simulink model "sl_groundvehicleDynamics"  (R2025a)
settings: Solver=ode45  StartTime=0.0  StopTime=1500  RelTol=1e-5  EnableMultiTasking=on
InitFcn:
  | mdl_robot;
undefined symbols (not defined in the file or in its folder): robot, waypoints
libraries: simulink x4, mobileRoboticsLib x3, simulink_extras x2
settings Model: Creator=sriramn  LastModifiedBy=n10971327
settings SolverCC: ZeroCrossAlgorithm=Adaptive  AlgebraicLoopSolver=TrustRegion
settings DataIOCC: LimitDataPoints=on  SaveFormat=Array  ReturnWorkspaceOutputs=off
settings OptimizationCC: ReuseModelBlockBuffer=off  LifeSpan=inf
settings DebuggingCC: SolverPrmCheckMsg=warning  UnconnectedInputMsg=warning  UnconnectedOutputMsg=warning  UnconnectedLineMsg=warning  AllowSymbolicDim=off  SFUnexpectedBacktrackingDiag=warning  SFNoUnconditionalDefaultTransitionDiag=warning  SFExecutionAtInitializationDiag=none  ArithmeticOperatorsInVariantConditions=warning
settings HardwareCC: ProdBitPerPointer=32.0  ProdBitPerSizeT=32.0  ProdBitPerPtrDiffT=32.0  ProdLargestAtomicFloat=None  ProdIntDivRoundTo=Undefined  ProdEndianess=Unspecified  ProdWordSize=32.0  ProdHWDeviceType=32-bit Generic
settings ModelReferenceCC: EnableRefExpFcnMdlSchedulingChecks=on  ModelReferenceMinAlgLoopOccurrences=on  PropagateSignalLabelsOutOfModel=off
settings SFSimCC: SimUseLocalCustomCode=off  CustomCodeUndefinedFunction=UseInterfaceOnly
settings RTWCC: RTWUseLocalCustomCode=off  GPUComputeCapability=3.5
settings CodeAppCC: StateflowObjectComments=on
settings GRTTargetCC: TargetLangStandard=C89/C90 (ANSI)
settings ConfigComp: CovMetricSettings=dw  CovSaveCumulativeToWorkspaceVar=on  CovSaveSingleToWorkspaceVar=on  CovExternalEMLEnable=off  CovSFcnEnable=off
settings SimscapeCC: SimscapeNormalizeSystem=off
settings ConfigurationSet: Description=SimMechanics 2G
settings ExplorerConfigSet: InternalSimMechanicsExplorerSettings="<ExplorerConfiguration><canonicalview>planar_xy</canonicalview><AnimationSetting><BasePlaybackSpeed>1.0</BasePlaybackSpeed><PlaybackSpeedFactor>1.0</PlaybackSpeedFactor></AnimationSetting><TilePanel><TileInfo><Tiles Columns=\"1\" Count=\"1\" Rows=\"1\"><Column Left=\"2\" Weight=\"1\"/><Column Left=\"1628\"/><Row Top=\"2\" Weight=\"1\"/><Row Top=\"1072\"/><Tile Height=\"1\" Width=\"1\" X=\"0\" Y=\"0\"/></Tiles></TileInfo><SceneInfo><SceneViewer><BGColor><R>0.60000002384185791</R><G>0.60000002384185791</G><B>0.60000002384185791</B></BGColor><Camera><Position><X>0.22951840878551699</X><Y>0.32651610611526627</Y><Z>-0.27215421354393321</Z></Position><Center><X>-0.15775714411666431</X><Y>-0.15462825985839526</Y><Z>0.065702552916005602</Z></Center><Up><X>-0.56030137557930915</X><Y>0.72817587161684794</Y><Z>0.39474329445726858</Z></Up><Left>-0.21481383955700509</Left><Right>0.21481383955700509</Right><Bottom>-0.27569784609469139</Bottom><Top>0.27569784609469139</Top></Camera></SceneViewer></SceneInfo></TilePanel></ExplorerConfiguration>"

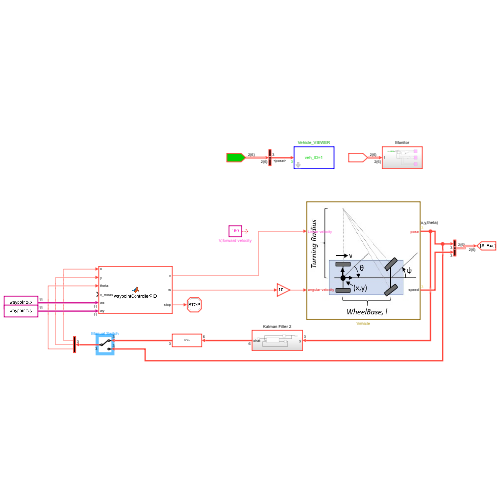
[thumbnail: Simulink's stored preview of the top-level diagram]
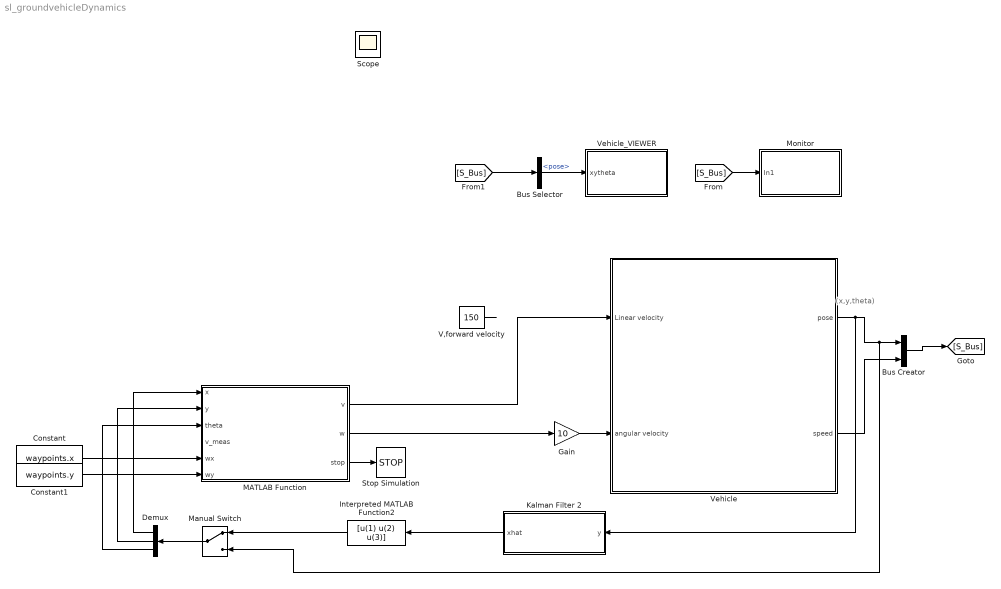
== system sl_groundvehicleDynamics ==
  note: (x,y,theta)
  Bus Creator : BusCreator  Inputs=2
  Bus Selector : BusSelector  OutputSignals=pose
  Constant : Constant  Value=waypoints.x
  Constant1 : Constant  Value=waypoints.y
  Demux : Demux  Outputs=3
  Gain : Gain  Gain=10
  Interpreted MATLAB Function2 : MATLABFcn  MATLABFcn=[u(1) u(2) u(3)]
  Kalman Filter 2 : Subsystem
  MATLAB Function : MATLAB Function  TreatAsAtomicUnit=on
  Manual Switch : ManualSwitch
  Monitor : Subsystem
  Stop Simulation : Stop
  V,forward velocity : Constant  Value=150
  Vehicle : Subsystem
      mask Display: image('vehicle.jpg');
  Vehicle_VIEWER : Subsystem  mask{wp_mat=[waypoints.x(:), waypoints.y(:)], veh_ID_num=1, veh_init_xytheta=[robot.X robot.Y robot.Theta], Ts=0.5}
      mask prompts: wp_mat "Waypoint matrix for arena [x_col, y_col] (m)"; veh_ID_num "Vehicle ID number"; veh_init_xytheta "Initial pose [x,y,theta]"; Ts "Sample time for updating animation (secs)"
      mask TypeOptions veh_ID_num: 1 | 2 | 3 | 4
      mask DialogControl Control2 Prompt: Animate simulation of Differential Drive Robot (DDR)
      mask Display: fprintf('veh_ID=%d',veh_ID_num);
  Scope : Scope
      settings: ActiveDisplayYMinimum=0.07  ActiveDisplayYMaximum=0.09
  wires:
  [S_Bus] -> Monitor/1(In1)
  [S_Bus] -> Bus Selector/1
  Vehicle/1(pose) -> Kalman Filter 2/1(y), Manual Switch/2, Bus Creator/1
  Vehicle/2(speed) -> Bus Creator/2
  Bus Creator/1 -> [S_Bus]
  Bus Selector/1 -> Vehicle_VIEWER/1(xytheta)  "<pose>"
  MATLAB Function/2(w) -> Gain/1
  V,forward velocity/1 -> ?
  Gain/1 -> Vehicle/2(angular velocity)
  MATLAB Function/3(stop) -> Stop Simulation/1
  Constant/1 -> MATLAB Function/5(wx)
  Constant1/1 -> MATLAB Function/6(wy)
  MATLAB Function/1(v) -> Vehicle/1(Linear velocity)
  Kalman Filter 2/1(xhat) -> Interpreted MATLAB Function2/1
  Demux/1 -> MATLAB Function/1(x)
  Interpreted MATLAB Function2/1 -> Manual Switch/1
  Manual Switch/1 -> Demux/1
  Demux/2 -> MATLAB Function/2(y)
  Demux/3 -> MATLAB Function/3(theta)

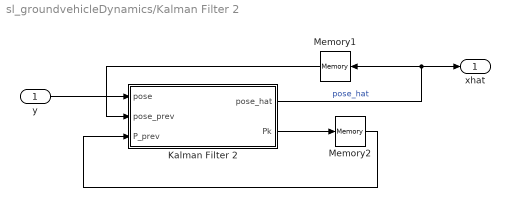
== system sl_groundvehicleDynamics/Kalman Filter 2 ==
  y : Inport
  Kalman Filter 2 : MATLAB Function  TreatAsAtomicUnit=on
  Memory1 : Memory  InheritSampleTime=on
  Memory2 : Memory  InheritSampleTime=on
  xhat : Outport
  wires:
  y/1 -> Kalman Filter 2/1(pose)
  Memory1/1 -> Kalman Filter 2/2(pose_prev)
  Kalman Filter 2/2(Pk) -> Memory2/1
  Kalman Filter 2/1(pose_hat) -> xhat/1, Memory1/1  "pose_hat"
  Memory2/1 -> Kalman Filter 2/3(P_prev)

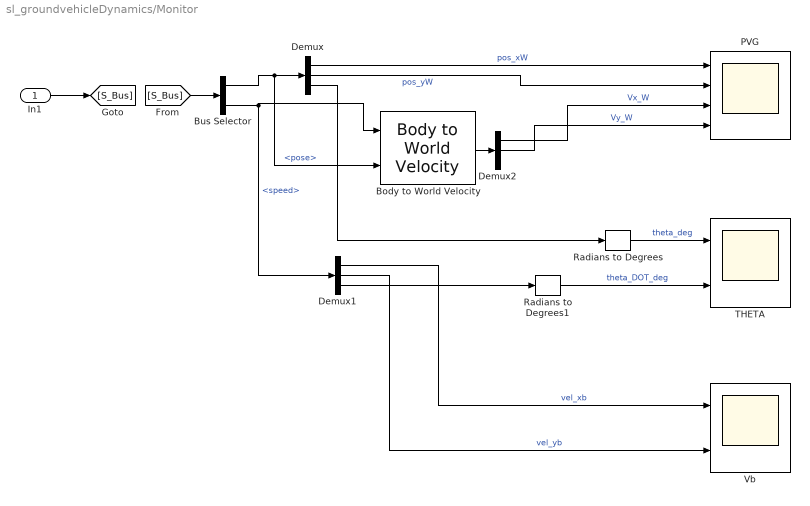
== system sl_groundvehicleDynamics/Monitor ==
  In1 : Inport
  Body to World Velocity : mobileRoboticsLib/Utilities/Body to World Velocity
      settings: SourceProductName=Mobile Robotics Simulation Toolbox
  Bus Selector : BusSelector  OutputSignals=pose,speed
  Demux : Demux  Outputs=3
  Demux1 : Demux  Outputs=3
  Demux2 : Demux  Outputs=3
  PVG : Scope  NumInputPorts=4
      settings: ActiveDisplayYMinimum=-3.02358  ActiveDisplayYMaximum=27.35477
  Radians to Degrees : simulink_extras/Transformations/Radians to Degrees
  Radians to Degrees1 : simulink_extras/Transformations/Radians to Degrees
  THETA : Scope  NumInputPorts=2
      settings: ActiveDisplayYMinimum=-8.72937  ActiveDisplayYMaximum=60.06611  DataLoggingVariableName=ScopeData2
  Vb : Scope  NumInputPorts=2
      settings: ActiveDisplayYMinimum=0.05577  ActiveDisplayYMaximum=0.8929
  wires:
  In1/1 -> [S_Bus]
  [S_Bus] -> Bus Selector/1
  Demux/1 -> PVG/1  "pos_xW"
  Demux/2 -> PVG/2  "pos_yW"
  Radians to Degrees1/1 -> THETA/2  "theta_DOT_deg"
  Radians to Degrees/1 -> THETA/1  "theta_deg"
  Demux1/3 -> Radians to Degrees1/1
  Demux/3 -> Radians to Degrees/1
  Bus Selector/1 -> Body to World Velocity/2, Demux/1  "<pose>"
  Bus Selector/2 -> Demux1/1, Body to World Velocity/1  "<speed>"
  Body to World Velocity/1 -> Demux2/1
  Demux2/1 -> PVG/3  "Vx_W"
  Demux2/2 -> PVG/4  "Vy_W"
  Demux1/1 -> Vb/1  "vel_xb"
  Demux1/2 -> Vb/2  "vel_yb"

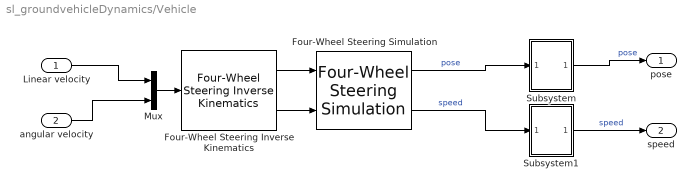
== system sl_groundvehicleDynamics/Vehicle ==
  Linear velocity : Inport
  angular velocity : Inport  Port=2
  Four-Wheel Steering Inverse Kinematics : mobileRoboticsLib/Kinematic Models/Four-Wheel Steering/Four-Wheel Steering Inverse Kinematics  wheelRadius=0.1  frontWheelDist=0.25  rearWheelDist=0.25  ikMode=Front Steering
      settings: SourceProductName=Mobile Robotics Simulation Toolbox
  Four-Wheel Steering Simulation : mobileRoboticsLib/Kinematic Models/Four-Wheel Steering/Four-Wheel Steering Simulation  wheelRadius=0.1  frontWheelDist=0.25  rearWheelDist=0.25  initX=robot.X  initY=robot.Y  initAngle=robot.Theta  Ts=0.05
      settings: SourceProductName=Mobile Robotics Simulation Toolbox
  Mux : Mux  Inputs=2
  Subsystem : Subsystem
  Subsystem1 : Subsystem
  pose : Outport  VectorParamsAs1DForOutWhenUnconnected=off
  speed : Outport  Port=2
  wires:
  angular velocity/1 -> Mux/2
  Linear velocity/1 -> Mux/1
  Mux/1 -> Four-Wheel Steering Inverse Kinematics/1
  Four-Wheel Steering Simulation/1 -> Subsystem/1(In1)  "pose"
  Four-Wheel Steering Simulation/2 -> Subsystem1/1(In1)  "speed"
  Four-Wheel Steering Inverse Kinematics/1 -> Four-Wheel Steering Simulation/1
  Four-Wheel Steering Inverse Kinematics/2 -> Four-Wheel Steering Simulation/2
  Subsystem/1(pose) -> pose/1  "pose"
  Subsystem1/1(speed) -> speed/1  "speed"

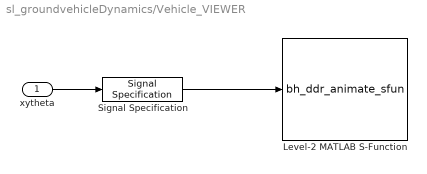
== system sl_groundvehicleDynamics/Vehicle_VIEWER ==
  xytheta : Inport
  Level-2 MATLAB S-Function : M-S-Function  FunctionName=bh_ddr_animate_sfun  Parameters=Ts, wp_mat, veh_ID_num, veh_init_xytheta
  Signal Specification : SignalSpecification  Dimensions=3
  wires:
  xytheta/1 -> Signal Specification/1
  Signal Specification/1 -> Level-2 MATLAB S-Function/1

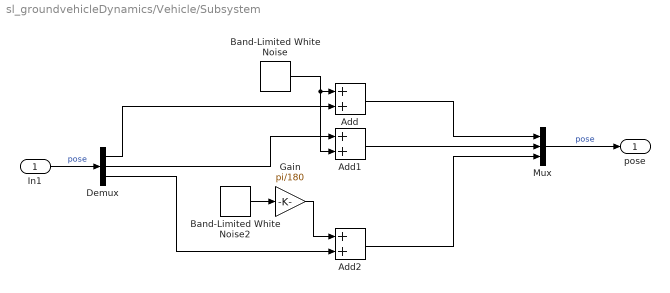
== system sl_groundvehicleDynamics/Vehicle/Subsystem ==
  In1 : Inport
  Add : Sum
  Add1 : Sum
  Add2 : Sum
  Band-Limited White Noise : simulink/Sources/Band-Limited White Noise  Cov=[0.001]  Ts=0.1  seed=[23341]
  Band-Limited White Noise2 : simulink/Sources/Band-Limited White Noise  Cov=[0.41]  Ts=0.1  seed=[23341]
  Demux : Demux  Outputs=3
  Gain : Gain  Gain=pi/180
  Mux : Mux  Inputs=3
  pose : Outport
  wires:
  Add1/1 -> Mux/2
  Add2/1 -> Mux/3
  Demux/2 -> Add1/1
  Band-Limited White Noise2/1 -> Gain/1
  Demux/3 -> Add2/2
  Band-Limited White Noise/1 -> Add1/2, Add/1
  In1/1 -> Demux/1  "pose"
  Demux/1 -> Add/2
  Gain/1 -> Add2/1
  Mux/1 -> pose/1  "pose"
  Add/1 -> Mux/1

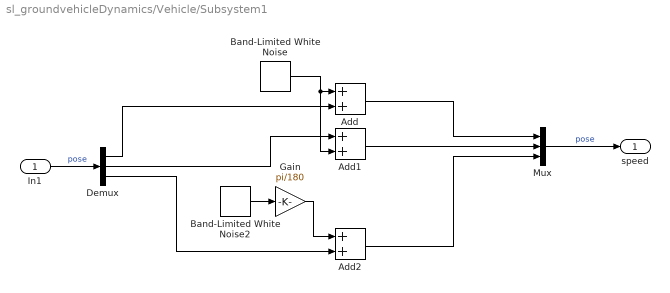
== system sl_groundvehicleDynamics/Vehicle/Subsystem1 ==
  In1 : Inport
  Add : Sum
  Add1 : Sum
  Add2 : Sum
  Band-Limited White Noise : simulink/Sources/Band-Limited White Noise  Cov=[0.001]  Ts=0.1  seed=[23341]
  Band-Limited White Noise2 : simulink/Sources/Band-Limited White Noise  Cov=[0.41]  Ts=0.1  seed=[23341]
  Demux : Demux  Outputs=3
  Gain : Gain  Gain=pi/180
  Mux : Mux  Inputs=3
  speed : Outport
  wires:
  Add1/1 -> Mux/2
  Add2/1 -> Mux/3
  Demux/2 -> Add1/1
  Band-Limited White Noise2/1 -> Gain/1
  Demux/3 -> Add2/2
  Band-Limited White Noise/1 -> Add1/2, Add/1
  In1/1 -> Demux/1  "pose"
  Demux/1 -> Add/2
  Gain/1 -> Add2/1
  Mux/1 -> speed/1  "pose"
  Add/1 -> Mux/1

== matlab function sl_groundvehicleDynamics/MATLAB Function ==
  data: v output; x input; w output; y input; theta input; v_meas input; wx input; wy input; stop output
function [v, w, stop] = waypointControllerPID(x, y, theta, v_meas, wx, wy)
%% Tuning Variables
% Controller sample time (s) – set to your model's controller step
Ts = 0.02;

% Heading PID (for w)
Kp_h = 1.6;     Ki_h = 0.20;   Kd_h = 0.05;
w_max = 1.2;                  % [rad/s] limit
i_lim_h = 2.0;                % integral clamp

% Speed PI (for v)
Kp_v = 1.0;     Ki_v = 0.5;
v_max = 100;   v_min = 0.0;   % [m/s]
i_lim_v = 5.0;

% Waypoint logic
capture_R   = 5.0;            % [m] switch waypoint
slow_R      = 40.0;           % [m] start slowing down near wp
e_slow_max  = pi/2;           % slow for big heading error (≈90°)

% Cruise bias (regular speed)
v_cruise    = 20;            % [m/s]
%% 

wx = wx(:);
wy = wy(:);
N  = numel(wx);

% Persistent state
persistent idx ih iv eh_prev Nprev
if isempty(idx);     idx = 1;        end
if isempty(ih);      ih  = 0.0;      end
if isempty(iv);      iv  = 0.0;      end
if isempty(eh_prev); eh_prev = 0.0;  end
if isempty(Nprev);   Nprev = N;      end

% Reset index if waypoint list size changed or index out of range
if (N ~= Nprev) || (idx < 1) || (idx > max(N,1))
    idx = 1;
    ih = 0.0; iv = 0.0; eh_prev = 0.0;
    Nprev = N;
end

% Default outputs
v = 0.0; w = 0.0; stop = 0;

% Guard empty waypoint list
if N == 0
    stop = 1;
    return;
end

% Current target waypoint
xw = wx(idx);  yw = wy(idx);

% Heading error (wrapped)
alpha = atan2(yw - y, xw - x);
eh    = wrapErr(alpha - theta);     % [-pi, pi]

% Distance to waypoint
d = hypot(x - xw, y - yw);

% --------- Speed scheduling (feedforward target) ----------
% Slow for big heading error
slow_heading   = clamp(1.0 - abs(eh)/e_slow_max, 0.0, 1.0);
% Slow as you approach the waypoint
slow_distance  = clamp(d/slow_R, 0.0, 1.0);
% Base desired speed
v_des = v_cruise * slow_heading * slow_distance;
v_des = clamp(v_des, v_min, v_max);

% --------- Heading PID -> angular rate w ------------------
ih = clamp(ih + eh*Ts, -i_lim_h, i_lim_h);    % integral
de = (eh - eh_prev) / max(Ts, 1e-6);          % derivative
w  = Kp_h*eh + Ki_h*ih + Kd_h*de;
w  = clamp(w, -w_max, w_max);
eh_prev = eh;

% --------- Speed PI -> forward speed v --------------------
ev = v_des - v_meas;
iv = clamp(iv + ev*Ts, -i_lim_v, i_lim_v);
v  = v_meas + Kp_v*ev + Ki_v*iv;              % absolute speed cmd
v  = clamp(v, v_min, v_max);

% --------- Waypoint switching & stop ----------------------
if d < capture_R
    if idx < N
        idx = idx + 1;
        % optional: clear heading integrator on wp switch
        ih = 0.0;
    else
        v = 0.0; w = 0.0;
        stop = 1;
    end
end

end

% ===== helpers =====
function z = clamp(x, a, b)
    z = min(max(x, a), b);
end

function e = wrapErr(x)
    % wrap to [-pi, pi]
    e = atan2(sin(x), cos(x));
end

== matlab function sl_groundvehicleDynamics/Kalman Filter 2/Kalman Filter 2 ==
  data: pose_hat output double size=6 [0..50]; pose input size=3 [0..50]; pose_prev input [0..50]; Pk output; P_prev input
function [pose_hat, Pk] = kalman_filter(pose, pose_prev, P_prev)

persistent first_entry
persistent counter
persistent x_hat
coder.extrinsic('disp');


% Initial state value
x0  = [0,0,0,0,0,0]';
xkh = x0;
Pk  = zeros(6,6);

if isempty(first_entry)
    first_entry = 0;  
end

if isempty(x_hat)
    x_hat= 0;  
end

if isempty(counter)
    counter = 0;  
end

dt       = 0.01;
pose_hat = pose_prev;
Pk       = P_prev;

sigma    = 1e-4;
sigmadot = sigma;
R        = 1.5;

A=[1,0,0,dt,0,0;...
   0,1,0,0,dt,0;...
   0,0,1,0,0,dt;...
   0,0,0,1,0,0;...
   0,0,0,0,1,0;
   0,0,0,0,0,1];


H = [ 1, 0, 0, 0, 0, 0 ; ...
      0, 1, 0, 0, 0, 0;...
      0, 0, 1, 0, 0, 0] ;
Q=diag([sigma,sigma,sigmadot,sigmadot,sigmadot,sigmadot]);
R=R*eye(3);



if first_entry == 0
  xkh = x0;
  Pk = 1000*eye(6);
  disp('initial')
end
% xkh
% Pk
% if(length(pose_hat)==6)
  xkh = pose_prev;
% end

% time update
xkhm=A*xkh;
Pkm=A*Pk*A'+ Q;

% measurement update
    Kk=Pkm*H'/(H*Pkm*H'+R);
    xkh=xkhm+Kk*(pose-H*xkhm);
    Pk=(eye(6)-Kk*H)*Pkm;
% store state estimates
    xkhat=xkh;

if first_entry == 0
    counter = 0;
    first_entry = 1;
end

counter = counter + 1;


for i=1:6
  pose_hat(i)=xkhat(i);
end
